simulink model "zad71_kaskada"  (R2015a)
settings: Solver=FixedStepDiscrete  StartTime=0.0  StopTime=99.0  FixedStep=1  RelTol=1e-3
settings Model: Creator=Bojana Vasic  LastModifiedBy=Bojana Vasic

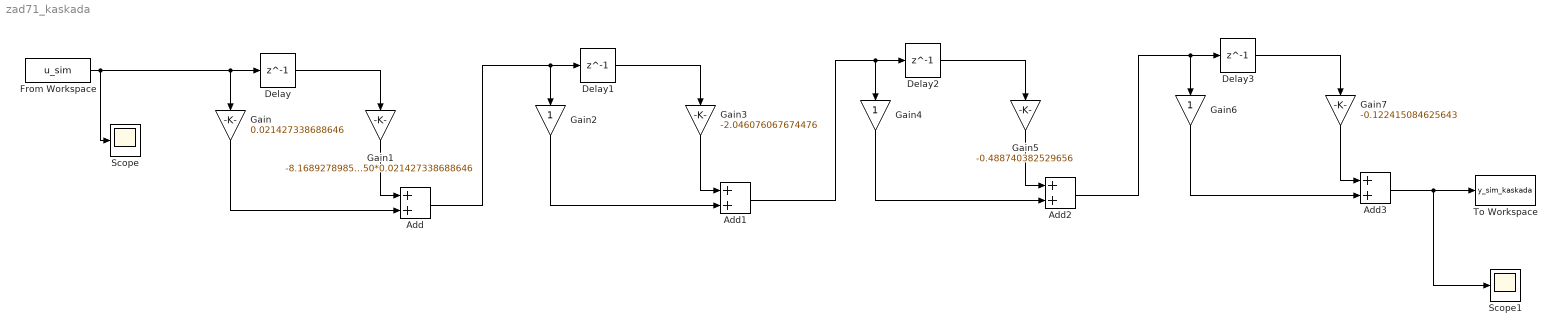
== system zad71_kaskada ==
  Add{,1..3} (4 alike) : Sum
  Delay{,1..3} (4 alike) : Delay  DelayLength=1
  From Workspace : FromWorkspace  VariableName=u_sim  SampleTime=1
  Gain : Gain  Gain=0.021427338688646
  Gain1 : Gain  Gain=-8.168927898535550*0.021427338688646
  Gain2 : Gain
  Gain3 : Gain  Gain=-2.046076067674476
  Gain4 : Gain
  Gain5 : Gain  Gain=-0.488740382529656
  Gain6 : Gain
  Gain7 : Gain  Gain=-0.122415084625643
  Scope : Scope
  Scope1 : Scope
  To Workspace : ToWorkspace  VariableName=y_sim_kaskada  SampleTime=-1
      settings: Save2DSignal=2-D array (concatenate along first dimension)
  wires:
  From Workspace/1 -> Scope/1, Gain/1, Delay/1
  Gain/1 -> Add/2
  Gain1/1 -> Add/1
  Delay/1 -> Gain1/1
  Add/1 -> Gain2/1, Delay1/1
  Gain2/1 -> Add1/2
  Gain3/1 -> Add1/1
  Delay1/1 -> Gain3/1
  Gain4/1 -> Add2/2
  Gain5/1 -> Add2/1
  Delay2/1 -> Gain5/1
  Add2/1 -> Gain6/1, Delay3/1
  Gain6/1 -> Add3/2
  Gain7/1 -> Add3/1
  Delay3/1 -> Gain7/1
  Add1/1 -> Gain4/1, Delay2/1
  Add3/1 -> To Workspace/1, Scope1/1
